simulink model "XBee Power Simulation"  (R2021b)
settings: Solver=VariableStepAuto  StartTime=0.0  StopTime=0.0005  MaxStep=1e-4  RelTol=1e-4  EnableMultiTasking=on
undefined symbols (not defined in the file): Hydride, Metal, Nickel
libraries: spsSeriesRLCBranchLib x8, spsVoltageMeasurementLib x3, spsCurrentMeasurementLib x2, spsACVoltageSourceLib x1, spsBatteryLib x1, spsDiodeLib x1, spsGroundLib x1, spsMosfetLib x1, spsPWMGeneratorDCDCLib x1, spspowerguiLib x1
settings Model: SimulationMode=accelerator  Creator=The MathWorks, Inc.  LastModifiedBy=Vivian Doan
settings SolverCC: AlgebraicLoopSolver=TrustRegion  SolverResetMethod=Robust
settings OptimizationCC: EfficientFloat2IntCast=on  LifeSpan=inf
settings DebuggingCC: ReadBeforeWriteMsg=DisableAll  WriteAfterWriteMsg=DisableAll  WriteAfterReadMsg=DisableAll  UniqueDataStoreMsg=error  StrictBusMsg=ErrorOnBusTreatedAsVector  SFUnexpectedBacktrackingDiag=warning  SFNoUnconditionalDefaultTransitionDiag=warning  SFExecutionAtInitializationDiag=none  SFMachineParentedDataDiag=warning  ArithmeticOperatorsInVariantConditions=warning
settings ModelReferenceCC: UpdateModelReferenceTargets=IfOutOfDate
settings SFSimCC: SFSimEcho=off  SimUseLocalCustomCode=off  CustomCodeUndefinedFunction=UseInterfaceOnly
settings RTWCC: RTWUseLocalCustomCode=off
settings CodeAppCC: StateflowObjectComments=on
settings GRTTargetCC: TargetLangStandard=C89/C90 (ANSI)
settings ConfigComp: CovMetricSettings=dw  CovSaveCumulativeToWorkspaceVar=on  CovSaveSingleToWorkspaceVar=on  CovExternalEMLEnable=off
settings SimscapeCC: SimscapeNormalizeSystem=off  SimscapeNominalValues={1, 'bar'; 1, 'cm^3/s'; 1, 'bar*kg/s'; 1, 'kJ/kg'; 1, 'kW'; }

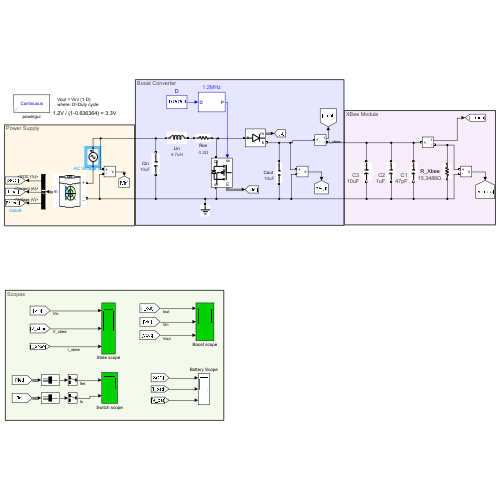
[thumbnail: Simulink's stored preview of the top-level diagram]
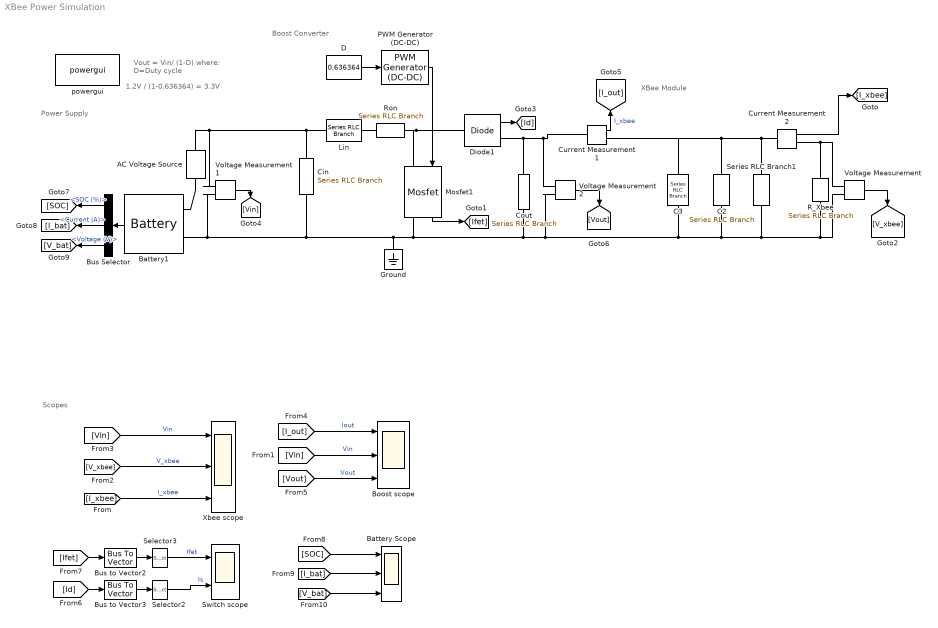
== system XBee Power Simulation ==
  note: Scopes
  note: XBee Module
  note: Boost Converter
  note: Power Supply
  note: 1.2V / (1-0.636364) = 3.3V
  note: Vout = Vin/ (1-D)
      | where: D=Duty cycle
  AC Voltage Source : spsACVoltageSourceLib/AC Voltage Source  Amplitude=0.9  Phase=0  Frequency=1.2e6  SampleTime=0  Measurements=None  BusType=swing  Pref=10e3  Qref=0  Qmin=-inf  Qmax=+inf
  Battery Scope : Scope  NumInputPorts=3
  Battery1 : spsBatteryLib/Battery  BatType=Nickel-Metal-Hydride  ShowTempParam=off  ThermalPreset=no  ShowAgeParam=off  NomV=1.2  NomQ=2.6  SOC=100  Batt_Tr=30  PresetModel=on  MaxQ=2.8  MinV=0.9  FullV=1.4136  Dis_rate=0.52  R=0.0046154  Normal_OP=2.5  expZone="[1.3017        0.52]"  current=[6.5 13 32.5]  Units=Time  Tci=20  NomT=20  T2=-30  MaxQ2=4.8  FullV2=7.1  Normal_OP2=5.655  expZone2="[6.58           1]"  Rca=0.6  ti=2000  Dp=0  Neq0=0  Tsim=1e6  Ta1=25  Qeol=5.4*0.9  Reol=0.013333*1.2  Char_age=[2.3478, 3]  Dis_age=[2.3478, 10]  N1=1500  N2=10500  N3=1000  N4=1400  Ta2=45  N5=950
  Boost scope : Scope  NumInputPorts=3
  Bus Selector : BusSelector  OutputSignals=SOC (%),Current (A),Voltage (V)
  Bus to Vector2 : BusToVector
  Bus to Vector3 : BusToVector
  C2 : spsSeriesRLCBranchLib/Series RLC Branch  LConnTagsString=__new0  RConnTagsString=__new0  BranchType=C  Resistance=1e-4  Inductance=200e-6  SetiL0=off  InitialCurrent=0  Capacitance=1e-6  Setx0=off  InitialVoltage=40  Measurements=None
      settings: AttributesFormatString=|
      | C2
      | 1uF
  C3 : spsSeriesRLCBranchLib/Series RLC Branch  LConnTagsString=__new0  RConnTagsString=__new0  BranchType=C  Resistance=1e-4  Inductance=200e-6  SetiL0=off  InitialCurrent=0  Capacitance=10e-6  Setx0=off  InitialVoltage=40  Measurements=None
      settings: AttributesFormatString=|
      | C3
      | 10uF
  Cin : spsSeriesRLCBranchLib/Series RLC Branch  LConnTagsString=__new0  RConnTagsString=__new0  BranchType=C  Resistance=1e-3  Inductance=4.7e-6  SetiL0=off  InitialCurrent=0  Capacitance=10e-6  Setx0=off  InitialVoltage=0  Measurements=None
      settings: AttributesFormatString=10uF
  Cout : spsSeriesRLCBranchLib/Series RLC Branch  LConnTagsString=__new0  RConnTagsString=__new0  BranchType=C  Resistance=1e-3  Inductance=4.7e-6  SetiL0=off  InitialCurrent=0  Capacitance=10e-6  Setx0=off  InitialVoltage=0  Measurements=None
      settings: AttributesFormatString=10uF
  Current Measurement1 : spsCurrentMeasurementLib/Current Measurement  PhasorSimulation=off  OutputType=Complex  PSBequivalent=0
  Current Measurement2 : spsCurrentMeasurementLib/Current Measurement  PhasorSimulation=off  OutputType=Complex  PSBequivalent=0
  D : Constant  Value=0.636364
  Diode1 : spsDiodeLib/Diode  Ron=1e-3  Lon=0  Vf=0  IC=0  UseSnubber=off  Rs=inf  Cs=inf  Measurements=on
  Ground : spsGroundLib/Ground  LConnTagsString=a
  Lin : spsSeriesRLCBranchLib/Series RLC Branch  LConnTagsString=__new0  RConnTagsString=__new0  BranchType=L  Resistance=0.3  Inductance=4.7e-6  SetiL0=off  InitialCurrent=0  Capacitance=1e-6  Setx0=off  InitialVoltage=0  Measurements=None
      settings: AttributesFormatString=4.7uH
  Mosfet1 : spsMosfetLib/Mosfet  Ron=1e-3  Lon=0  Rd=1e-3  Vfd=0  IC=0  Rs=inf  Cs=inf  Measurements=on
  PWM Generator (DC-DC) : spsPWMGeneratorDCDCLib/PWM Generator (DC-DC)  Fsw=1.2e6  Ts=0
      settings: AttributesFormatString=1.2MHz
  R_Xbee : spsSeriesRLCBranchLib/Series RLC Branch  LConnTagsString=__new0  RConnTagsString=__new0  BranchType=R  Resistance=15.3488  Inductance=200e-6  SetiL0=off  InitialCurrent=0  Capacitance=400e-6  Setx0=off  InitialVoltage=0  Measurements=None
      settings: AttributesFormatString=15.3488Ω
  Ron : spsSeriesRLCBranchLib/Series RLC Branch  LConnTagsString=__new0  RConnTagsString=__new0  BranchType=R  Resistance=0.3  Inductance=4.7e-6  SetiL0=off  InitialCurrent=0  Capacitance=1e-6  Setx0=off  InitialVoltage=0  Measurements=None
      settings: AttributesFormatString=0.3Ω
  Selector2 : Selector  InputPortWidth=2  IndexOptions=Index vector (dialog)  Indices=1  OutputSizes=1
  Selector3 : Selector  InputPortWidth=2  IndexOptions=Index vector (dialog)  Indices=1  OutputSizes=1
  Series RLC Branch1 : spsSeriesRLCBranchLib/Series RLC Branch  LConnTagsString=__new0  RConnTagsString=__new0  BranchType=C  Resistance=1e-4  Inductance=200e-6  SetiL0=off  InitialCurrent=0  Capacitance=47e-12  Setx0=off  InitialVoltage=40  Measurements=None
      settings: AttributesFormatString=|
      | C1
      | 47pF
  Switch scope : Scope  NumInputPorts=2
  Voltage Measurement : spsVoltageMeasurementLib/Voltage Measurement  PhasorSimulation=off  OutputType=Complex  PSBequivalent=0
  Voltage Measurement1 : spsVoltageMeasurementLib/Voltage Measurement  PhasorSimulation=off  OutputType=Complex  PSBequivalent=0
  Voltage Measurement2 : spsVoltageMeasurementLib/Voltage Measurement  PhasorSimulation=off  OutputType=Complex  PSBequivalent=0
  Xbee scope : Scope  NumInputPorts=3
  powergui : spspowerguiLib/powergui  Priority=1  SimulationMode=Continuous  SampleTime=50e-6  frequency=60  Iterations=50  frequencyindice=0  Pbase=100e6  ErrMax=1e-4  UnitsV=kV  UnitsW=MW  buscounter=0  FunctionMessages=off  echomessages=off  EnableUseOfTLC=off  CurrentSourceSwitches=off  DisableSnubberDevices=off  DisableRonSwitches=off  DisableVfSwitches=off  DisplayEquations=off  AutomaticDiscreteSolvers=off  SolverType=Tustin/Backward Euler (TBE)  Interpol=off  ExternalGateDelay=off  methode=off  Ts=100  x0status=blocks  SPID=on  SwTol=0  HookPort=off  NonlinearTolerance=1e-4  nMaxIteration=100  ContinueOnMaxIteration=off  RestoreLinks=warning  ResistiveCurrentMeasurement=off  Frange=[0:2:500]  Ylog=off  Xlog=on  ShowGrid=off  save=off  variable=ZData  structure=0  ZoomFFT=off  StartTime=0.0  cycles=1  DisplayStyle=1  fundamental=60  FreqAxis=off  MaxFrequency=1000  frequencyindicesteady=1  RmsSteady=1  display=off
  wires:
  Voltage Measurement/1 -> [V_xbee]
  Mosfet1/1 -> [Ifet]
  Diode1/1 -> [Id]
  PWM Generator (DC-DC)/1 -> Mosfet1/1
  D/1 -> PWM Generator (DC-DC)/1
  Voltage Measurement1/1 -> [Vin]
  [Vin] -> Boost scope/2  "Vin"
  Battery1/1 -> Bus Selector/1
  Bus Selector/2 -> [I_bat]  "<Current (A)>"
  Current Measurement2/1 -> [I_xbee]
  [V_xbee] -> Xbee scope/2  "V_xbee"
  [Vin] -> Xbee scope/1  "Vin"
  [I_xbee] -> Xbee scope/3  "I_xbee"
  Current Measurement1/1 -> [I_out]  "I_xbee"
  [I_out] -> Boost scope/1  "Iout"
  Voltage Measurement2/1 -> [Vout]
  [Vout] -> Boost scope/3  "Vout"
  [Ifet] -> Bus to Vector2/1
  Bus to Vector2/1 -> Selector3/1
  Selector3/1 -> Switch scope/1  "Ifet"
  [Id] -> Bus to Vector3/1
  Bus to Vector3/1 -> Selector2/1
  Selector2/1 -> Switch scope/2  "Is"
  Bus Selector/1 -> [SOC]  "<SOC (%)>"
  Bus Selector/3 -> [V_bat]  "<Voltage (V)>"
  [SOC] -> Battery Scope/1
  [I_bat] -> Battery Scope/2
  [V_bat] -> Battery Scope/3
  connections:
  R_Xbee/RConn1 -- C2/RConn1 -- C3/RConn1 -- Voltage Measurement2/LConn2 -- Cout/RConn1 -- Ground/LConn1 -- Cin/RConn1 -- Voltage Measurement1/LConn2 -- Battery1/LConn2 -- Mosfet1/RConn1 -- Series RLC Branch1/RConn1 -- Voltage Measurement/LConn2
  Diode1/RConn1 -- Voltage Measurement2/LConn1 -- Current Measurement1/LConn1 -- Cout/LConn1
  Lin/LConn1 -- Cin/LConn1 -- Voltage Measurement1/LConn1 -- AC Voltage Source/RConn1
  Mosfet1/LConn1 -- Ron/RConn1 -- Diode1/LConn1
  AC Voltage Source/LConn1 -- Battery1/LConn1
  Voltage Measurement/LConn1 -- R_Xbee/LConn1 -- Current Measurement2/RConn1
  Current Measurement2/LConn1 -- Current Measurement1/RConn1 -- C3/LConn1 -- C2/LConn1 -- Series RLC Branch1/LConn1
  Lin/RConn1 -- Ron/LConn1
